simulink subsystem "BEV1EMSSC"  (R2023a)
settings: Solver=VariableStepAuto  StartTime=0.0  StopTime=10.0  RelTol=1e-3
libraries: fl_lib x3, nesl_utility_internal x1
settings Model: Creator=The MathWorks, Inc.  LastModifiedBy=The MathWorks, Inc.
settings OptimizationCC: ReuseModelBlockBuffer=off
settings DebuggingCC: SubsystemReferenceDiagnosticForUnitTest=warning

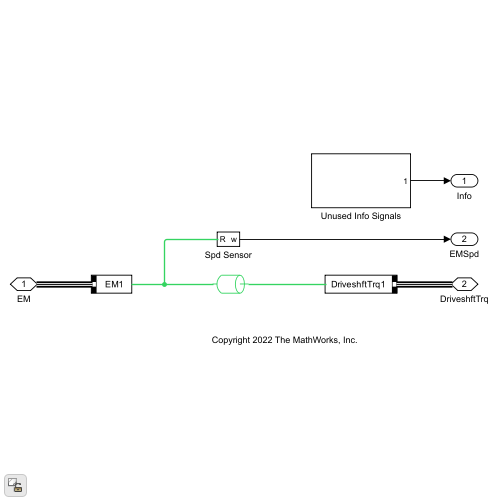
[thumbnail: Simulink's stored preview of the top-level diagram]
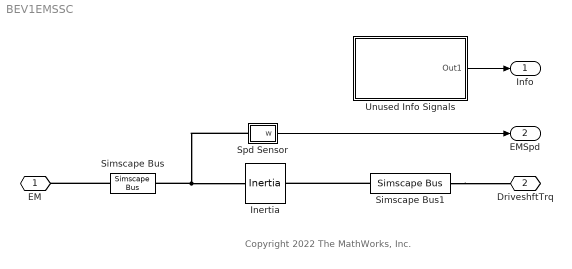
== system BEV1EMSSC ==
  note: Copyright 2022 The MathWorks, Inc.
  Inertia : fl_lib/Mechanical/Rotational Elements/Inertia  inertia=PlntEM1RotInertia kg*m^2  num_ports=foundation.enum.numPorts2.two  w_specify=off  w_priority=High  w=0 rad/s  w_nominal_specify=off  w_nominal_unit=rad/s  w_nominal_value=1  t_specify=off  t_priority=None  t=0 N*m  t_nominal_specify=off  t_nominal_unit=N*m  t_nominal_value=1
      settings: InternalSimscapePortConfiguration="{\"Bottom\":[],\"Left\":[{\"id\":\"I\",\"label\":\"\",\"type\":\"foundation.mechanical.rotational.rotational\"}],\"Right\":[{\"id\":\"J\",\"label\":\"\",\"type\":\"foundation.mechanical.rotational.rotational\"}],\"Top\":[]}"
  Simscape Bus : SimscapeBus  HierarchyStrings=EM1
  Simscape Bus1 : SimscapeBus  HierarchyStrings=DriveshftTrq1
  Spd Sensor : Subsystem
  Unused Info Signals : Subsystem
  EM : PMIOPort  Side=Left
  DriveshftTrq : PMIOPort  Port=2  Side=Right
  Info : Outport  VectorParamsAs1DForOutWhenUnconnected=off  BusOutputAsStruct=on
  EMSpd : Outport  Port=2  VectorParamsAs1DForOutWhenUnconnected=off  BusOutputAsStruct=on
  wires:
  Spd Sensor/1(w) -> EMSpd/1
  Unused Info Signals/1(Out1) -> Info/1
  connections:
  Spd Sensor/LConn1 -- Inertia/RConn1 -- Simscape Bus/LConn1
  Simscape Bus/RConn1 -- EM/RConn1
  Simscape Bus1/RConn1 -- DriveshftTrq/RConn1
  Simscape Bus1/LConn1 -- Inertia/LConn1

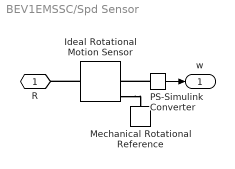
== system BEV1EMSSC/Spd Sensor ==
  Ideal Rotational Motion Sensor : fl_lib/Mechanical/Mechanical Sensors/Ideal Rotational Motion Sensor  reference=foundation.enum.MeasurementReference.difference  acceleration_port=false  velocity_port=true  position_port=true  wrap_angle=simscape.enum.onoff.off  offset=0 rad
  Mechanical Rotational Reference : fl_lib/Mechanical/Rotational Elements/Mechanical Rotational Reference
  PS-Simulink Converter : nesl_utility_internal/PS-Simulink Converter  PhysicalDomain=network_engine_domain  SubClassName=ps_output  LeftPortType=input  RightPortType=output  PseudoPeriodic=off  Frequencies=[]  VectorFormat=inherit  Unit=inherit  AffineConversion=off
  R : PMIOPort  Side=Left
  w : Outport
  wires:
  PS-Simulink Converter/1 -> w/1
  connections:
  Ideal Rotational Motion Sensor/RConn1 -- Mechanical Rotational Reference/LConn1
  Ideal Rotational Motion Sensor/LConn1 -- R/RConn1
  PS-Simulink Converter/LConn1 -- Ideal Rotational Motion Sensor/RConn2

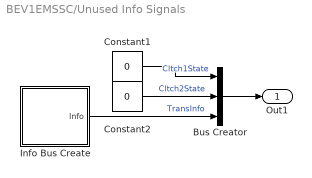
== system BEV1EMSSC/Unused Info Signals ==
  Bus Creator : BusCreator  Inputs=3
  Constant1 : Constant  Value=0  SampleTime=-1
  Constant2 : Constant  Value=0  SampleTime=-1
  Info Bus Create : Subsystem
  Out1 : Outport
  wires:
  Constant2/1 -> Bus Creator/2  "Cltch2State"
  Constant1/1 -> Bus Creator/1  "Cltch1State"
  Bus Creator/1 -> Out1/1
  Info Bus Create/1(Info) -> Bus Creator/3  "TransInfo"

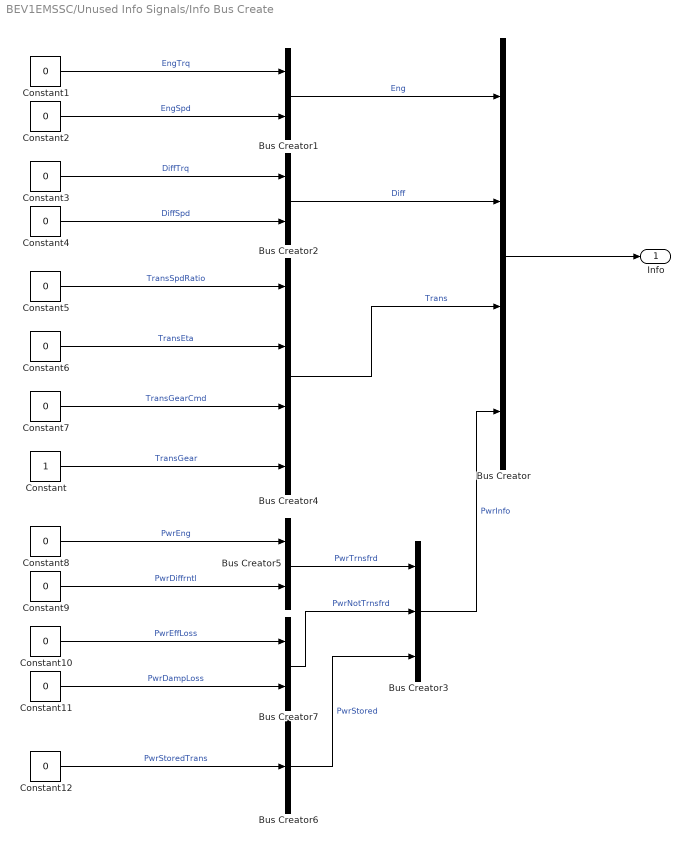
== system BEV1EMSSC/Unused Info Signals/Info Bus Create ==
  Bus Creator : BusCreator  Inputs=4
  Bus Creator{1..2,5,7} (4 alike) : BusCreator  Inputs=2
  Bus Creator3 : BusCreator  Inputs=3
  Bus Creator4 : BusCreator  Inputs=4
  Bus Creator6 : BusCreator  Inputs=1
  Constant : Constant  SampleTime=-1
  Constant{1..12} (12 alike) : Constant  Value=0  SampleTime=-1
  Info : Outport
  wires:
  Bus Creator5/1 -> Bus Creator3/1  "PwrTrnsfrd"
  Bus Creator6/1 -> Bus Creator3/3  "PwrStored"
  Bus Creator7/1 -> Bus Creator3/2  "PwrNotTrnsfrd"
  Constant12/1 -> Bus Creator6/1  "PwrStoredTrans"
  Bus Creator2/1 -> Bus Creator/2  "Diff"
  Constant9/1 -> Bus Creator5/2  "PwrDiffrntl"
  Constant7/1 -> Bus Creator4/3  "TransGearCmd"
  Constant10/1 -> Bus Creator7/1  "PwrEffLoss"
  Constant1/1 -> Bus Creator1/1  "EngTrq"
  Constant5/1 -> Bus Creator4/1  "TransSpdRatio"
  Bus Creator/1 -> Info/1
  Constant3/1 -> Bus Creator2/1  "DiffTrq"
  Constant11/1 -> Bus Creator7/2  "PwrDampLoss"
  Constant/1 -> Bus Creator4/4  "TransGear"
  Constant2/1 -> Bus Creator1/2  "EngSpd"
  Bus Creator1/1 -> Bus Creator/1  "Eng"
  Constant6/1 -> Bus Creator4/2  "TransEta"
  Constant4/1 -> Bus Creator2/2  "DiffSpd"
  Constant8/1 -> Bus Creator5/1  "PwrEng"
  Bus Creator3/1 -> Bus Creator/4  "PwrInfo"
  Bus Creator4/1 -> Bus Creator/3  "Trans"
